simulink model "oven_pwm"  (Simulink 7.4)
settings: Solver=ode45  StartTime=0.0  StopTime=60*30  MaxStep=0.01  RelTol=1e-3
libraries: powerlib_extras x1
settings Model: Creator=psonna  LastModifiedBy=psonna

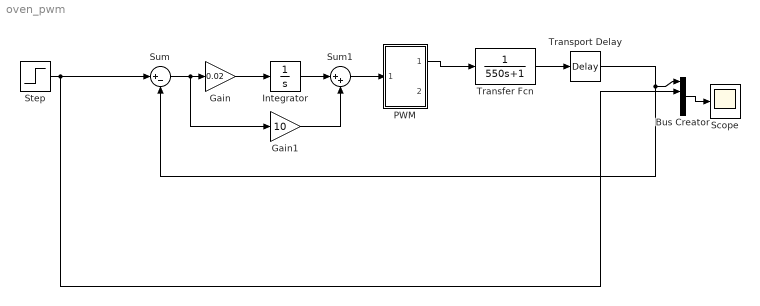
== system oven_pwm ==
  Bus Creator : BusCreator
  Gain : Gain  Gain=0.02  ParameterDataType=fixdt(1, 16)  ParameterScaling=2^0  OutDataType=fixdt(1, 16)  OutScaling=2^0
  Gain1 : Gain  Gain=10  ParameterDataType=fixdt(1, 16)  ParameterScaling=2^0  OutDataType=fixdt(1, 16)  OutScaling=2^0
  Integrator : Integrator
  PWM : Subsystem
  Scope : Scope
      settings: YMin=0  YMax=0.0012
  Step : Step  After=0.001  SampleTime=0
  Sum : Sum  Inputs=|+-  OutDataType=fixdt(1, 16)  OutScaling=2^0
  Sum1 : Sum  Inputs=|++  OutDataType=fixdt(1, 16)  OutScaling=2^0
  Transfer Fcn : TransferFcn  Denominator=[550 1]
  Transport Delay : TransportDelay  DelayTime=36
  wires:
  Transfer Fcn/1 -> Transport Delay/1
  Step/1 -> Bus Creator/2, Sum/1
  Bus Creator/1 -> Scope/1
  Transport Delay/1 -> Bus Creator/1, Sum/2
  Sum/1 -> Gain/1, Gain1/1
  PWM/1(Out1) -> Transfer Fcn/1
  Gain/1 -> Integrator/1
  Integrator/1 -> Sum1/1
  Sum1/1 -> PWM/1(In1)
  Gain1/1 -> Sum1/2

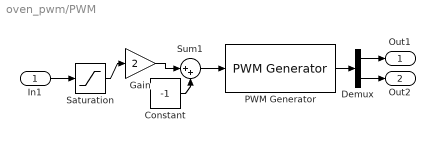
== system oven_pwm/PWM ==
  In1 : Inport
  Constant : Constant  Value=-1  OutDataType=fixdt(1, 16)  OutScaling=2^0
  Demux : Demux  Outputs=2
  Gain : Gain  Gain=2  ParameterDataType=fixdt(1, 16)  ParameterScaling=2^0  OutDataType=fixdt(1, 16)  OutScaling=2^0
  PWM Generator : powerlib_extras/Control  Blocks/PWM Generator  DialogController=POWERSYS.PowerSysDialog  SystemSampleTime=-1  GeneratorMode="1-arm  bridge (2 pulses)"  Fc=0.1  Internal=off  mIndex=0.4  Freq=60  Phase=0
  Saturation : Saturate  OutDataType=fixdt(1, 16)  OutScaling=2^0
  Sum1 : Sum  Inputs=|++  OutDataType=fixdt(1, 16)  OutScaling=2^0
  Out1 : Outport
  Out2 : Outport  Port=2
  wires:
  PWM Generator/1 -> Demux/1
  Sum1/1 -> PWM Generator/1
  Saturation/1 -> Gain/1
  Constant/1 -> Sum1/2
  Gain/1 -> Sum1/1
  Demux/1 -> Out1/1
  Demux/2 -> Out2/1
  In1/1 -> Saturation/1
